simulink model "async_simulink_control_client_2024a"  (R2024a)
settings: Solver=ode4  StartTime=0.0  StopTime=100  FixedStep=0.5  RelTol=1e-3
settings Model: Creator=yaozhong.zhang  LastModifiedBy=Admin
settings SolverCC: AlgebraicLoopSolver=TrustRegion
settings DebuggingCC: UnconnectedInputMsg=warning  UnconnectedOutputMsg=warning  UnconnectedLineMsg=warning
settings ModelReferenceCC: EnableRefExpFcnMdlSchedulingChecks=on
settings RTWCC: GPUComputeCapability=3.5

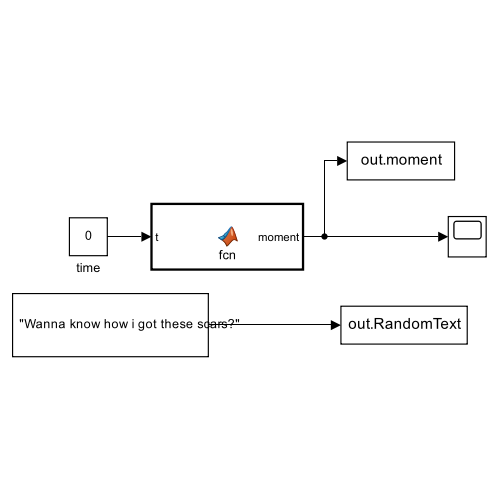
[thumbnail: Simulink's stored preview of the top-level diagram]
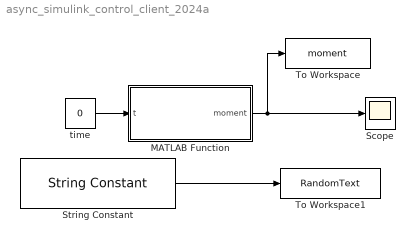
== system async_simulink_control_client_2024a ==
  MATLAB Function : MATLAB Function  TreatAsAtomicUnit=on
  Scope : Scope
  String Constant : StringConstant  String="\"Wanna know how i got these scars?\""
  To Workspace : ToWorkspace  VariableName=moment  SampleTime=-1
      settings: Save2DSignal=2-D array (concatenate along first dimension)
  To Workspace1 : ToWorkspace  VariableName=RandomText  SaveFormat=Timeseries  SampleTime=-1
  time : Constant  Value=0  SampleTime=-1
  wires:
  MATLAB Function/1(moment) -> To Workspace/1, Scope/1
  time/1 -> MATLAB Function/1(t)
  String Constant/1 -> To Workspace1/1

== matlab function async_simulink_control_client_2024a/MATLAB Function ==
  data: t input; moment output
function moment = fcn(t)
if floor(mod(t, 2))
    moment = 20;
else
    moment = 5;
end
